simulink model "slcontrolbeam"  (R2023a)
settings: Solver=ode45  StartTime=0  StopTime=50  MaxStep=0.4  RelTol=1e-3  AbsTol=1e-6
PreLoadFcn:
  | tank=readfis('tank');
values from neighbouring files (symbols this model uses):
  g = 9.85    [Beam_Parameters.m]    (also in animballandbeam.m = 0.05)
  J = 1/12*mb*L^2    (= 0.16875)    [Beam_Parameters.m]
  L = 3    [Beam_Parameters.m]
  m = 0.1    [Beam_Parameters.m]
  R = 0.15    [Beam_Parameters.m]
libraries: fuzblock x1, simulink_need_slupdate x1
CloseFcn:
  | AnimFigH = findobj(0,'Name', 'Tank Demo'); close(AnimFigH)
settings Model: PacingRate=1000  Creator=pascal  LastModifiedBy=marco
settings SolverCC: AutoScaleAbsTol=off  ZeroCrossAlgorithm=Adaptive  AlgebraicLoopSolver=TrustRegion
settings DataIOCC: SaveFormat=Array  SignalLoggingSaveFormat=ModelDataLogs  SaveOutput=off  SaveTime=off  ReturnWorkspaceOutputs=off
settings OptimizationCC: BlockReduction=off  BooleanDataType=off  ExpressionDepthLimit=2147483647  InitFltsAndDblsToZero=on  LifeSpan=inf
settings DebuggingCC: SaveWithParameterizedLinksMsg=none  UnderspecifiedInitializationDetection=Classic  MergeDetectMultiDrivingBlocksExec=none  SignalResolutionControl=TryResolveAllWithWarning  IgnoredZcDiagnostic=none  MultiTaskDSMMsg=warning  MultiTaskCondExecSysMsg=none  FcnCallInpInsideContextMsg=warning  UnconnectedInputMsg=warning  UnconnectedOutputMsg=warning  UnconnectedLineMsg=warning  StateNameClashWarn=warning  SFUnexpectedBacktrackingDiag=warning  SFNoUnconditionalDefaultTransitionDiag=warning  SFExecutionAtInitializationDiag=none  ArithmeticOperatorsInVariantConditions=warning
settings HardwareCC: ProdBitPerPointer=32  ProdBitPerSizeT=32  ProdBitPerPtrDiffT=32  ProdLargestAtomicFloat=None  ProdIntDivRoundTo=Undefined  ProdEndianess=Unspecified  ProdWordSize=32  ProdHWDeviceType=32-bit Generic  TargetBitPerPointer=64  TargetBitPerSizeT=64  TargetBitPerPtrDiffT=64  TargetLongLongMode=on  TargetIntDivRoundTo=Zero  TargetEndianess=LittleEndian  TargetWordSize=64  TargetHWDeviceType=MATLAB Host  ProdEqTarget=off
settings ModelReferenceCC: EnableRefExpFcnMdlSchedulingChecks=on  PropagateSignalLabelsOutOfModel=off
settings SFSimCC: SimUseLocalCustomCode=off  CustomCodeUndefinedFunction=UseInterfaceOnly
settings RTWCC: GenerateMakefile=off  TemplateMakefile=grt_unix.tmf  RTWUseLocalCustomCode=off
settings CodeAppCC: StateflowObjectComments=on
settings GRTTargetCC: TargetFcnLib=ansi_tfl_tmw.mat  TargetLangStandard=C89/C90 (ANSI)  CombineOutputUpdateFcns=off  GRTInterface=on
settings ConfigComp: CovMetricSettings=dw  CovSaveCumulativeToWorkspaceVar=on  CovSaveSingleToWorkspaceVar=on  CovExternalEMLEnable=off

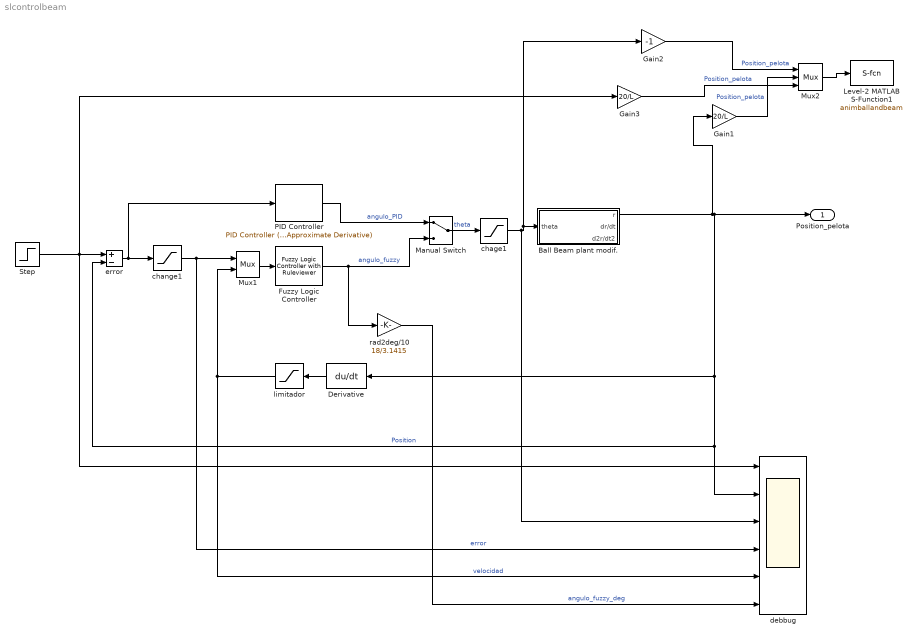
== system slcontrolbeam ==
  Ball Beam plant modif. : Subsystem
  Derivative : Derivative  CoefficientInTFapproximation=100000000
  "Fuzzy Logic Controller " : fuzblock/Fuzzy Logic  Controller  with Ruleviewer  fismatrix=FCbeam_30_reglas_v2  Ts=5
  Gain1 : Gain  Gain=20/L
  Gain2 : Gain  Gain=-1
  Gain3 : Gain  Gain=20/L
  Level-2 MATLAB S-Function1 : M-S-Function  FunctionName=animballandbeam  Parameters=1
  Manual Switch : ManualSwitch
  Mux1 : Mux  Inputs=2
  Mux2 : Mux  Inputs=3
  PID Controller : simulink_need_slupdate/PID Controller (with Approximate Derivative)  P=8  I=0.01  D=15  N=1000
  Step : Step  SampleTime=0
  chage1 : Saturate  UpperLimit=0.2617  LowerLimit=-0.2617
  change1 : Saturate  UpperLimit=1  LowerLimit=-1
  debbug : Scope  NumInputPorts=6
  error : Sum  Inputs=+-  InputSameDT=on  SaturateOnIntegerOverflow=on  OutDataTypeStr=Inherit: Same as first input
  limitador : Saturate  UpperLimit=0.1  LowerLimit=-0.1
  rad2deg/10 : Gain  Gain=18/3.1415
  Position_pelota : Outport
  wires:
  Derivative/1 -> limitador/1
  Mux1/1 -> "Fuzzy Logic Controller "/1
  limitador/1 -> debbug/5, Mux1/2  "velocidad"
  PID Controller/1 -> Manual Switch/1  "angulo_PID"
  "Fuzzy Logic Controller "/1 -> Manual Switch/2, rad2deg/10/1  "angulo_fuzzy"
  change1/1 -> debbug/4, Mux1/1  "error"
  error/1 -> change1/1, PID Controller/1
  rad2deg/10/1 -> debbug/6  "angulo_fuzzy_deg"
  Ball Beam plant modif./1(r) -> Gain1/1, Position_pelota/1, debbug/2, error/2, Derivative/1  "Position"
  Step/1 -> Gain3/1, debbug/1, error/1
  Mux2/1 -> Level-2 MATLAB S-Function1/1
  Gain1/1 -> Mux2/2  "Position_pelota"
  Gain2/1 -> Mux2/1  "Position_pelota"
  Gain3/1 -> Mux2/3  "Position_pelota"
  Manual Switch/1 -> chage1/1  "theta"
  chage1/1 -> debbug/3, Gain2/1, Ball Beam plant modif./1(theta)

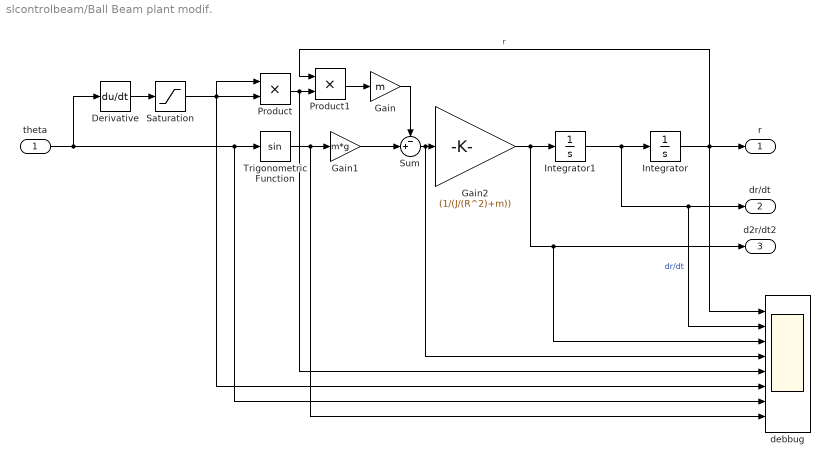
== system slcontrolbeam/Ball Beam plant modif. ==
  theta : Inport
  Derivative : Derivative  CoefficientInTFapproximation=1000
  Gain : Gain  Gain=m
  Gain1 : Gain  Gain=m*g
  Gain2 : Gain  Gain=(1/(J/(R^2)+m))
  Integrator : Integrator
  Integrator1 : Integrator
  Product : Product
  Product1 : Product
  Saturation : Saturate  LinearizeAsGain=off  ZeroCross=off
  Sum : Sum  Inputs=-+|
  Trigonometric Function : Trigonometry
  debbug : Scope  NumInputPorts=8
  r : Outport
  dr/dt : Outport  Port=2
  d2r/dt2 : Outport  Port=3
  wires:
  Derivative/1 -> Saturation/1
  Integrator1/1 -> debbug/2, dr/dt/1, Integrator/1  "dr/dt"
  Integrator/1 -> debbug/1, Product1/1, r/1  "r"
  theta/1 -> debbug/7, Trigonometric Function/1, Derivative/1
  Gain2/1 -> debbug/3, d2r/dt2/1, Integrator1/1
  Product/1 -> debbug/5, Product1/2
  Product1/1 -> Gain/1
  Sum/1 -> debbug/4, Gain2/1
  Trigonometric Function/1 -> debbug/8, Gain1/1
  Gain1/1 -> Sum/2
  Gain/1 -> Sum/1
  Saturation/1 -> Product/1, debbug/6, Product/2
